simulink model "MTU_HVM_5_0a"  (Simulink 7.7)
settings: Solver=ode23  StartTime=0.0  StopTime=TEST_CYCLE(end,1)  FixedStep=0.01  RelTol=1e-3
InitFcn:
  | Vehicle_Init_File
values from neighbouring files (symbols this model uses):
  Batt_Aux_Load_W = 800    [Student_Design_Parameters.m]
  Engine_ACC_Loss_Nm = 4.6    [ICE_Tech_Specs.m]
  Engine_BSFC_2DMAP_g_kWh = Engine_BSFC_2DMAP_g_kWh'    [ICE_Tech_Specs.m]    (also in Student_Design_Parameters.m = 1.00*Engine_BSFC_2DMAP_g_kWh)
  Engine_Max_Speed_rpm = 6800    [ICE_Tech_Specs.m]
  Engine_Min_Speed_rpm = 600    [ICE_Tech_Specs.m]
  Engine_Startup_Fuel_g = 4.0*Engine_Displacement_L/3.6    (= 2.66666666667)    [ICE_Tech_Specs.m]
  Engine_Torque_2DMAP_Nm = Engine_Torque_2DMAP_Nm'    [ICE_Tech_Specs.m]
  Motor_Gear_Ratio = 1.00    (= 1)    [Student_Design_Parameters.m]
  Motor_Km = 0.94    [Motor_Tech_Specs.m]
  Motor_Ra = 0.106    [Motor_Tech_Specs.m]
  Motor_Torque_Peak_Nm = T    [Motor_Tech_Specs.m]
  Motor_Torque_Speed_Index_rpm = N    [Motor_Tech_Specs.m]
  TEST_CYCLE = [0 1 2 3 4 5 6 7 8 9 10 11 ... (1900 elements, 950x2)]    [Constant_Speed_Points_Cycle.mat]    (also in US06_Cycle.mat = [0 1 2 3 4 5 6 7 8 9 10 11 ... (1202 elements, 601x2)])
  TRANS_Differential_Ratio = 3.25    [Student_Design_Parameters.m]
  TRANS_DS_THRES = 1.0*TRANS_DS_THRES    [Student_Design_Parameters.m]
  TRANS_US_THRES = 1.0*TRANS_US_THRES    [Student_Design_Parameters.m]
  Vehicle_Drag_Coeff = F2/(0.5*Air_Density_kgm*Vehicle_Frontal_Area_m)    [Student_Design_Parameters.m]
  Vehicle_Frontal_Area_m = h*w*0.0254*0.0254    [Student_Design_Parameters.m]
  Vehicle_Mass_kg = 1549    [Student_Design_Parameters.m]
  Vehicle_Tire_Coeff_Rolling_Resistance = 0.008    [Student_Design_Parameters.m]
  Vehicle_Tire_Radius_m = 0.95*26.311/2*0.0254    (= 0.317442215)    [Student_Design_Parameters.m]
undefined symbols (not defined in the file or in its folder): Air_Density_kgm, Batt_a, Batt_Capacity_Ah, Batt_Const_V, Batt_dG, Batt_Disable_SOC, Batt_Initial_SOC, Batt_Lower_Volt_Limit_V, Batt_Max_Charge_Current_A, Batt_Max_Discharge_Current_A, Batt_Max_SOC, Batt_Min_SOC, Batt_Numb_Cells_N, Batt_OCV_Z, Batt_Resis_Ohms, Batt_Upper_Volt_Limit_V, Batt_Warburg_Capcitance_F, Batt_Warburg_Resis_Ohms, Fuel_Density_kgm3, Gravity, Max_Vehicle_Speed_Control_Error_mph, TRANS_Gear_Ratio, Vehicle_Tire_Rolling_Fric_Velocity_Modifier, Vehicle_Tire_Static_Fric_Coeff, Vehicle_Tractive_Force_Limit
libraries: simulink x8
(part 2 of 2)

== system MTU_HVM_5_0a/Electric Motor/PMDC Electrical ==
  "Motor Speed, rads1" : Inport
  Motor Torque NM : Inport  Port=2
  1/Km : Gain  Gain=1/Motor_Km
  Add2 : Sum
  Km1 : Gain  Gain=Motor_Km
  Ra1 : Gain  Gain=Motor_Ra
  "Motor Current, A1" : Outport
  "Motor Voltage, V1" : Outport  Port=2
  wires:
  "Motor Speed, rads1"/1 -> Km1/1
  Motor Torque NM/1 -> 1/Km/1
  Km1/1 -> Add2/1  "Ea"
  Ra1/1 -> Add2/2
  Add2/1 -> "Motor Voltage, V1"/1
  1/Km/1 -> "Motor Current, A1"/1, Ra1/1  "ia"

== system MTU_HVM_5_0a/Electric Motor/PMDC Mechanical ==
  "Motor Speed, rads" : Inport
  Normalized Motor Torque Request : Inport  Port=2
  Product2 : Product  RndMeth=Zero
  Speed vs Torque : Lookup  InputValues=Motor_Torque_Speed_Index_rpm  Table=Motor_Torque_Peak_Nm  LookUpMeth=Interpolation-Use End Values
  rad/s to rpm : Gain  Gain=30/3.14159
  "Motor Torque, Nm" : Outport
  wires:
  [Motor_Speed_rpm] -> Speed vs Torque/1
  "Motor Speed, rads"/1 -> rad/s to rpm/1
  rad/s to rpm/1 -> [Motor_Speed_rpm]
  Normalized Motor Torque Request/1 -> [Motor_Torque_Request]
  [Motor_Torque_Request] -> Product2/1
  Speed vs Torque/1 -> Product2/2
  Product2/1 -> "Motor Torque, Nm"/1

== system MTU_HVM_5_0a/Electric Motor/Power Electronics ==
  "Battery Voltage, V1" : Inport
  "Motor Voltage, V1" : Inport  Port=2
  "Motor Current, A1" : Inport  Port=3
  Add1 : Sum
  Mult1 : Product  Inputs=/*
  Mult2 : Product  Inputs=**
  Ron1 : Gain  Gain=0.01
  Saturation : Saturate  UpperLimit=inf  LowerLimit=1
  "Battery Current, A" : Outport
  wires:
  "Motor Current, A1"/1 -> Ron1/1, Mult2/2
  "Battery Voltage, V1"/1 -> Saturation/1
  Saturation/1 -> Mult1/1
  "Motor Voltage, V1"/1 -> Add1/1
  Ron1/1 -> Add1/2
  Add1/1 -> Mult1/2  "Vab"
  Mult1/1 -> Mult2/1  "Duty Cycle"
  Mult2/1 -> "Battery Current, A"/1

== system MTU_HVM_5_0a/LVD/If Action Subsystem ==
  In1 : Inport
  Action Port : ActionPort  ActionType=then
  Out1 : Outport
  wires:
  In1/1 -> Out1/1

== system MTU_HVM_5_0a/LVD/If Action Subsystem1 ==
  In1 : Inport
  Action Port : ActionPort  ActionType=else
  Out1 : Outport
  wires:
  In1/1 -> Out1/1

== system MTU_HVM_5_0a/LVD/Sign + Logic to have Rolling resitance =0 N when Velocity=0 mps ==
  note: Added in version 3.1b
      | to fix zero speed issue
  note: Better to implement as gain /
      | saturation block to avoid
      | discontinuities
  Velocity_mps : Inport
  Abs1 : Abs
  Constant1 : Constant  Value=0
  Constant4 : Constant
  Product : Product  RndMeth=Zero
  Sign : Signum  ZeroCross=off
  Switch : Switch  Criteria=u2 > Threshold  Threshold=1e-4
  Sign with zero logic : Outport
  wires:
  Abs1/1 -> Switch/2
  Velocity_mps/1 -> Abs1/1, Sign/1
  Constant4/1 -> Switch/1
  Constant1/1 -> Switch/3
  Switch/1 -> Product/2
  Product/1 -> Sign with zero logic/1
  Sign/1 -> Product/1

== system MTU_HVM_5_0a/LVD/Sign(V)*V^2 ==
  Velocity (m/s) : Inport
  Math Function : Math  Operator=square  SaturateOnIntegerOverflow=on
  Product : Product  RndMeth=Zero
  Sign : Signum  ZeroCross=off
  sign(V)*V^2 : Outport
  wires:
  Velocity (m/s)/1 -> Math Function/1, Sign/1
  Math Function/1 -> Product/1
  Sign/1 -> Product/2
  Product/1 -> sign(V)*V^2/1

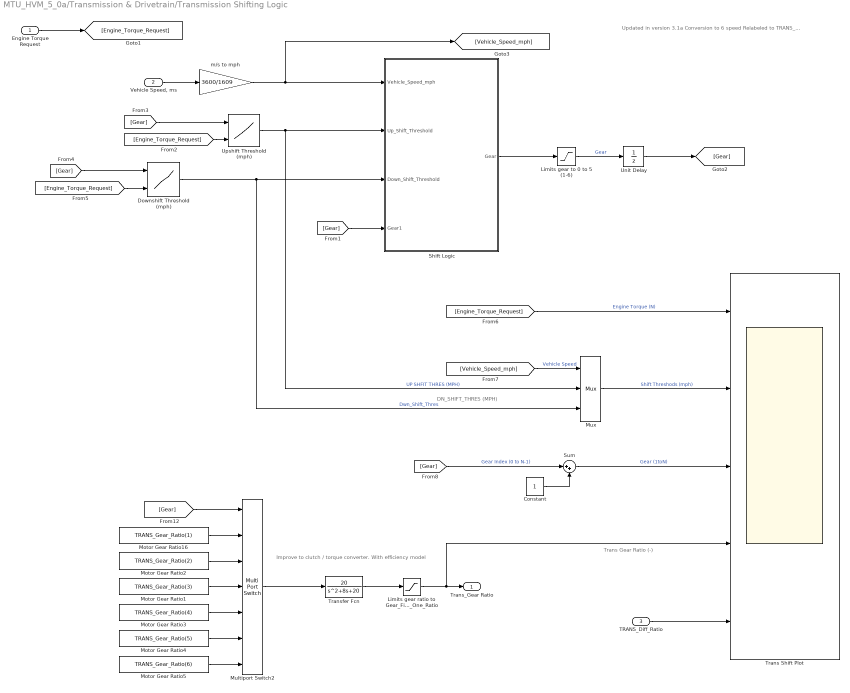
== system MTU_HVM_5_0a/Transmission & Drivetrain/Transmission Shifting Logic ==
  note: DN_SHIFT_THRES (MPH)
  note: Updated in version 3.1a
      | Conversion to 6 speed
      | Relabeled to TRANS_...
  note: Improve to clutch / torque converter.
      | With efficiency model
  note: Trans Gear Ratio (-)
  Engine Torque Request : Inport
  "Vehicle Speed, ms" : Inport  Port=2
  TRANS_Diff_Ratio : Inport  Port=3
  Constant : Constant
  Downshift Threshold (mph) : Lookup2D  RowIndex=TRANS_GEAR_INDEX  ColumnIndex=TRANS_TORQUE_INDEX  Table=TRANS_DS_THRES  LookUpMeth=Interpolation-Use End Values
  Limits gear ratio to Gear_Five_Ratio to Gear_One_Ratio : Saturate  UpperLimit=TRANS_Gear_Ratio(1)  LowerLimit=TRANS_Gear_Ratio(end)
  Limits gear to 0 to 5 (1-6) : Saturate  UpperLimit=5  LowerLimit=0
  Motor Gear Ratio1 : Constant  Value=TRANS_Gear_Ratio(3)
  Motor Gear Ratio16 : Constant  Value=TRANS_Gear_Ratio(1)
  Motor Gear Ratio2 : Constant  Value=TRANS_Gear_Ratio(2)
  Motor Gear Ratio3 : Constant  Value=TRANS_Gear_Ratio(4)
  Motor Gear Ratio4 : Constant  Value=TRANS_Gear_Ratio(5)
  Motor Gear Ratio5 : Constant  Value=TRANS_Gear_Ratio(6)
  Multiport Switch2 : MultiPortSwitch  DataPortOrder=Zero-based contiguous  Inputs=6  zeroidx=on
  Mux : Mux  Inputs=3
  Shift Logic : Stateflow chart  TreatAsAtomicUnit=on
  Sum : Sum  Inputs=|++
  Trans Shift Plot : Scope  NumInputPorts=5
      settings: Description=Diagnostics Plot for Transmission Shifting  YMin=0~-25~3~-5~-5  YMax=1~150~4~5~5  SaveName=Diagnostics_Trans_Shifting  SampleInput=on  SampleTime=0.1
  Transfer Fcn : TransferFcn  Numerator=20  Denominator=[1 8 20]
  Unit Delay : UnitDelay  SampleTime=-1
  Upshift Threshold (mph) : Lookup2D  RowIndex=TRANS_GEAR_INDEX  ColumnIndex=TRANS_TORQUE_INDEX  Table=TRANS_US_THRES  LookUpMeth=Interpolation-Use End Values
  m/s to mph : Gain  Gain=3600/1609
  Trans_Gear Ratio : Outport
  wires:
  "Vehicle Speed, ms"/1 -> m/s to mph/1
  Engine Torque Request/1 -> [Engine_Torque_Request]
  Limits gear ratio to Gear_Five_Ratio to Gear_One_Ratio/1 -> Trans_Gear Ratio/1, Trans Shift Plot/4
  [Engine_Torque_Request] -> Downshift Threshold (mph)/2
  [Gear] -> Downshift Threshold (mph)/1
  [Engine_Torque_Request] -> Upshift Threshold (mph)/2
  [Gear] -> Upshift Threshold (mph)/1
  Upshift Threshold (mph)/1 -> Shift Logic/2(Up_Shift_Threshold), Mux/2  "UP SHFIT THRES (MPH)"
  m/s to mph/1 -> Shift Logic/1(Vehicle_Speed_mph), [Vehicle_Speed_mph]
  [Gear] -> Multiport Switch2/1
  Motor Gear Ratio16/1 -> Multiport Switch2/2
  Motor Gear Ratio1/1 -> Multiport Switch2/4
  Motor Gear Ratio3/1 -> Multiport Switch2/5
  Motor Gear Ratio4/1 -> Multiport Switch2/6
  Multiport Switch2/1 -> Transfer Fcn/1
  Limits gear to 0 to 5 (1-6)/1 -> Unit Delay/1  "Gear"
  Transfer Fcn/1 -> Limits gear ratio to Gear_Five_Ratio to Gear_One_Ratio/1
  Shift Logic/1(Gear) -> Limits gear to 0 to 5 (1-6)/1
  [Gear] -> Shift Logic/4(Gear1)
  Unit Delay/1 -> [Gear]
  [Engine_Torque_Request] -> Trans Shift Plot/1  "Engine Torque (N)"
  [Vehicle_Speed_mph] -> Mux/1  "Vehicle Speed"
  Mux/1 -> Trans Shift Plot/2  "Shift Threshods (mph)"
  Downshift Threshold (mph)/1 -> Shift Logic/3(Down_Shift_Threshold), Mux/3  "Dwn_Shift_Thres"
  [Gear] -> Sum/1  "Gear Index (0 to N-1)"
  Constant/1 -> Sum/2
  Sum/1 -> Trans Shift Plot/3  "Gear (1toN)"
  Motor Gear Ratio5/1 -> Multiport Switch2/7
  Motor Gear Ratio2/1 -> Multiport Switch2/3
  TRANS_Diff_Ratio/1 -> Trans Shift Plot/5

== matlab function Transmission & Drivetrain/Transmission Shifting Logic/Shift Logic ==
  data: Vehicle_Speed_mph input double; Gear output double; Up_Shift_Threshold input double; Down_Shift_Threshold input double; Gear1 input double
function Gear = fcn(Vehicle_Speed_mph, Up_Shift_Threshold,...
    Down_Shift_Threshold, Gear1)
% This block supports the Embedded MATLAB subset.
% See the help menu for details.


if Vehicle_Speed_mph < 5
    Gear = 0;
elseif Vehicle_Speed_mph >= Up_Shift_Threshold
    Gear = Gear1 + 1;
elseif Vehicle_Speed_mph <= Down_Shift_Threshold
    Gear = Gear1 - 1;
else
    Gear = Gear1;
end

Gear = max(0, Gear);

== matlab function Electric Motor/Embedded MATLAB Function ==
  data: Motor_Torque_Request input double; Flag output double; Battery_SOC input double; Max_Battery_SOC input double; Min_Battery_SOC input double
function Flag = fcn(Motor_Torque_Request,Battery_SOC,Max_Battery_SOC,Min_Battery_SOC)
%#eml
if(Motor_Torque_Request<0 && Battery_SOC>=Max_Battery_SOC)
    Flag=0;
elseif(Motor_Torque_Request>0 && Battery_SOC<=Min_Battery_SOC)
    Flag=0;
else
    Flag=1;
end
